simulink model "OMAP_ver_MIL10"  (R2018b)
settings: Solver=FixedStepDiscrete  StartTime=0.0  StopTime=10.0  FixedStep=0.01  RelTol=1e-3
undefined symbols (not defined in the file or in its folder): OMAP_Switch_EMS, OMAP_Switch_EPS, OMAP_Switch_ESC, OMAP_Switch_IC, OMAP_Switch_OTHER, TH_HMIClb_tiDgrdIconWarnHiDurT_C, TH_HMIClb_tiDgrdIconWarnLoDurT_C, TH_HMIClb_tiDgrdVocWarnDurT_C, TH_HMIClb_tiHndOffTxtWarnT_C, TH_HMIClb_tiHndOffVocWarnT_C, TH_HMIClb_tiSWALimFlgDetT_C, TH_HMIClb_tiTxtLimT_C
libraries: simulink x118
(part 4 of 9)

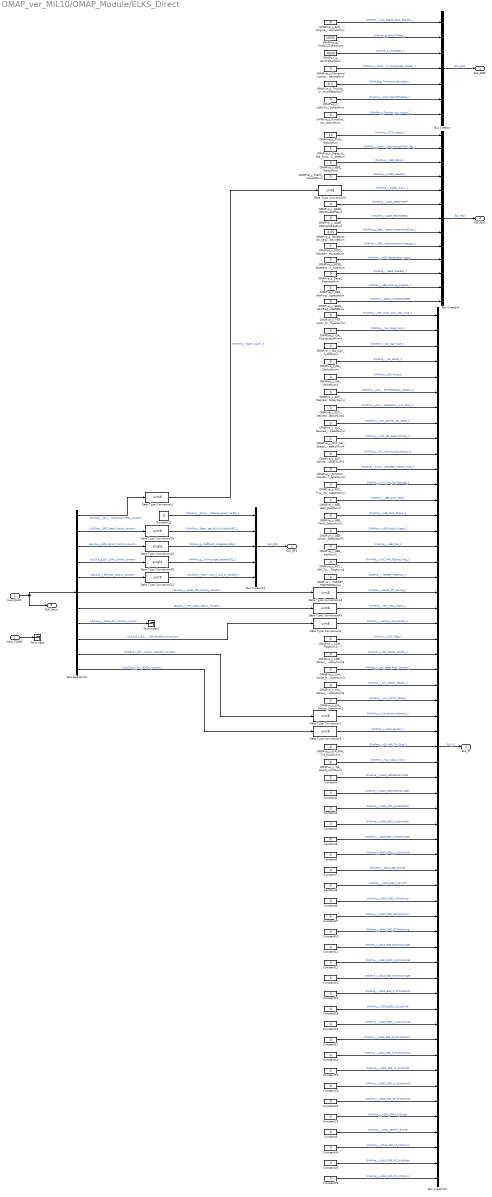
== system OMAP_ver_MIL10/OMAP_Module/ELKS_Direct ==
  Input_ELKS : Inport
  Input_FDMM : Inport  Port=2
  Bus Creator : BusCreator  Inputs=7
  Bus Creator13 : BusCreator  Inputs=5
  Bus Creator22 : BusCreator  Inputs=57
  Bus Creator5 : BusCreator  Inputs=13
  Bus Selector10 : BusSelector  OutputSignals=ELKSve_y_ELK_HapticAlarmReq_convert,ELKSve_y_EPS_State_Control_convert,ELKSve_g_EPS_Factor_Control_convert,ELKSve_g_ELK_SWA_Control_convert,ELKSve_y_EPS_ELK_Control_convert,ELKSve_y_Hands_Off_Warning_convert,ELKSve_y_HMI_Popup_Status_convert,ELKSve_y_state_ELK_function_convert,ELKSve_y_ELK_VehicleLaneDisp_convert,ELKSve_y_ELK_Action_Indication_convert,ELKSve_y_ELK_ELKSts_convert
  Constant{,1..27} (28 alike) : Constant  Value=0  OutDataTypeStr=uint8
  Data Type Conversion{1..5,28,31,44..45} (9 alike) : DataTypeConversion  OutDataTypeStr=uint8
  Data Type Conversion29 : DataTypeConversion  OutDataTypeStr=single
  Data Type Conversion30 : DataTypeConversion  OutDataTypeStr=single
  OMAPve_g_ACCTqReqNum : Constant  Value=-4000  OutDataTypeStr=single
  OMAPve_g_Deceleration_setpoint_deviceNum : Constant  Value=2.05  OutDataTypeStr=single
  OMAPve_g_PotACCTqReqNum : Constant  Value=-4000  OutDataTypeStr=single
  OMAPve_g_TminUp_or_downGearNum : Constant  Value=6.2  OutDataTypeStr=single
  OMAPve_y_ACC_DesiredHeadway_DisplayNum4 : Constant  Value=0  OutDataTypeStr=uint8
  OMAPve_y_ACC_DesiredHeadway_Icon_BasicNum4 : Constant  Value=0  OutDataTypeStr=uint8
  OMAPve_y_ACC_Desired_Set_SpeedNum4 : Constant  Value=0  OutDataTypeStr=uint8
  OMAPve_y_ACC_Engine_Start_RequestNum : Constant  Value=0  OutDataTypeStr=uint8
  OMAPve_y_ACC_HMI_TgtDisp_FlagNum4 : Constant  Value=0  OutDataTypeStr=uint8
  OMAPve_y_ACC_Pop_Up_MessageNum4 : Constant  Value=0  OutDataTypeStr=uint8
  OMAPve_y_ACC_Set_Speed_DisplayNum4 : Constant  Value=0  OutDataTypeStr=uint8
  OMAPve_y_ACC_Vehicle_Icon_DisplayNum4 : Constant  Value=0  OutDataTypeStr=uint8
  OMAPve_y_ADAS_ACCRequestEPBNum : Constant  Value=0  OutDataTypeStr=uint8
  OMAPve_y_ADAS_ESCDriveOffNum : Constant  Value=0  OutDataTypeStr=uint8
  OMAPve_y_ADAS_ESCHoldReqNum : Constant  Value=0  OutDataTypeStr=uint8
  OMAPve_y_AEB_Alert_ReqNum2 : Constant  Value=0  OutDataTypeStr=uint8
  OMAPve_y_AEB_Braking_progressNum : Constant  Value=0  OutDataTypeStr=uint8
  OMAPve_y_AEB_Fault_StatusNum2 : Constant  Value=0  OutDataTypeStr=uint8
  OMAPve_y_AEB_StatusNum : Constant  Value=5  OutDataTypeStr=uint8
  OMAPve_y_AEB_Switch_StatusNum2 : Constant  Value=0  OutDataTypeStr=uint8
  OMAPve_y_AEB_tipsNum2 : Constant  Value=0  OutDataTypeStr=uint8
  OMAPve_y_Decel_RequestNum : Constant  Value=0  OutDataTypeStr=uint8
  OMAPve_y_FCW_StatusNum : Constant  Value=10  OutDataTypeStr=uint8
  OMAPve_y_Function_Acc_statusNum : Constant  Value=3  OutDataTypeStr=uint8
  OMAPve_y_ICA_HMI_Txt_DispNum4 : Constant  Value=0  OutDataTypeStr=uint8
  OMAPve_y_ISA_Popup_textNum4 : Constant  Value=0  OutDataTypeStr=uint8
  OMAPve_y_ISA_Sign_TypeNum4 : Constant  Value=0  OutDataTypeStr=uint8
  OMAPve_y_ISA_StatusNum4 : Constant  Value=0  OutDataTypeStr=uint8
  OMAPve_y_ISA_ValueNum4 : Constant  Value=0  OutDataTypeStr=uint8
  OMAPve_y_LDW_FlagNum3 : Constant  Value=0  OutDataTypeStr=uint8
  OMAPve_y_LDW_Status_DisplayNum3 : Constant  Value=0  OutDataTypeStr=uint8
  OMAPve_y_LKA_Mode_from_CameraNum3 : Constant  Value=0  OutDataTypeStr=uint8
  OMAPve_y_LKA_Status_DisplayNum3 : Constant  Value=0  OutDataTypeStr=uint8
  OMAPve_y_LKA_Switch_StateNum3 : Constant  Value=0  OutDataTypeStr=uint8
  OMAPve_y_MDD_Decelerationcontrol_requestNum : Constant  Value=0  OutDataTypeStr=uint8
  OMAPve_y_MDD_deceleration_typeNum : Constant  Value=0  OutDataTypeStr=uint8
  OMAPve_y_Powertrain_torquewheel_requestNum : Constant  Value=0  OutDataTypeStr=uint8
  OMAPve_y_Prefill_requestNum : Constant  Value=0  OutDataTypeStr=uint8
  OMAPve_y_RVVACC_Vehiclespeed_request_typeNum4 : Constant  Value=0  OutDataTypeStr=uint8
  OMAPve_y_State_of_the_functionFARC_detNum : Constant  Value=5  OutDataTypeStr=uint8
  OMAPve_y_TARGET_POSITIONNum4 : Constant  Value=6  OutDataTypeStr=uint8
  OMAPve_y_TJA_status_iconNum4 : Constant  Value=0  OutDataTypeStr=uint8
  OMAPve_y_TSR_Vision_Only_Sign_TypeNum4 : Constant  Value=0  OutDataTypeStr=uint8
  OMAPve_y_stAcvTqWhlPTPotReqNum : Constant  Value=0  OutDataTypeStr=uint8
  Terminator : Terminator
  Terminator1 : Terminator
  ELK_EMS : Outport
  ELK_ESC : Outport  Port=2
  ELK_EPS : Outport  Port=3
  ELK_IC : Outport  Port=4
  ELK_Input : Outport  Port=5
  wires:
  Bus Creator22/1 -> ELK_IC/1  "ELK_IC"
  Data Type Conversion44/1 -> Bus Creator22/19  "OMAPve_y_Hands_off_warning_2"
  Data Type Conversion1/1 -> Bus Creator22/27  "OMAPve_y_LKA_action_indication_2"
  Bus Selector10/5 -> Data Type Conversion31/1  "<ELKSve_y_EPS_ELK_Control_convert>"
  Bus Selector10/2 -> Data Type Conversion28/1  "<ELKSve_y_EPS_State_Control_convert>"
  Data Type Conversion29/1 -> Bus Creator13/3  "OMAPve_g_Coefficient_toregulate_EPS_2"
  OMAPve_y_LDW_Status_DisplayNum3/1 -> Bus Creator22/23  "OMAPve_y_LDW_Status_Display_2"
  OMAPve_y_LDW_FlagNum3/1 -> Bus Creator22/22  "OMAPve_y_LDW_Flag_2"
  OMAPve_y_ACC_DesiredHeadway_Icon_BasicNum4/1 -> Bus Creator22/7  "OMAPve_y_ACC_DesiredHeadway_Icon_Basic_2"
  Bus Selector10/6 -> Data Type Conversion44/1  "<ELKSve_y_Hands_Off_Warning_convert>"
  Bus Selector10/4 -> Data Type Conversion30/1  "<ELKSve_g_ELK_SWA_Control_convert>"
  OMAPve_y_ACC_HMI_TgtDisp_FlagNum4/1 -> Bus Creator22/17  "OMAPve_y_ACC_HMI_TgtDisp_Flag_2"
  Bus Selector10/3 -> Data Type Conversion29/1  "<ELKSve_g_EPS_Factor_Control_convert>"
  Data Type Conversion4/1 -> Bus Creator22/21  "OMAPve_y_Vehicle_Lane_Display_2"
  OMAPve_y_TJA_status_iconNum4/1 -> Bus Creator22/30  "OMAPve_y_TJA_status_icon_2"
  Bus Selector10/8 -> Terminator1/1  "<ELKSve_y_state_ELK_function_convert>"
  OMAPve_y_TARGET_POSITIONNum4/1 -> Bus Creator22/18  "OMAPve_y_TARGET_POSITION_2"
  OMAPve_y_ACC_Vehicle_Icon_DisplayNum4/1 -> Bus Creator22/10  "OMAPve_y_ACC_Vehicle_Icon_Display_2"
  OMAPve_y_ACC_DesiredHeadway_DisplayNum4/1 -> Bus Creator22/6  "OMAPve_y_ACC_DesiredHeadway_Display_2"
  OMAPve_y_LKA_Status_DisplayNum3/1 -> Bus Creator22/25  "OMAPve_y_LKA_Status_Display_2"
  OMAPve_y_AEB_tipsNum2/1 -> Bus Creator22/16  "OMAPve_y_AEB_tips_2"
  OMAPve_y_ACC_Pop_Up_MessageNum4/1 -> Bus Creator22/12  "OMAPve_y_ACC_Pop_Up_Message_2"
  Bus Selector10/7 -> Data Type Conversion45/1  "<ELKSve_y_HMI_Popup_Status_convert>"
  OMAPve_y_ACC_Desired_Set_SpeedNum4/1 -> Bus Creator22/8  "OMAPve_y_ACC_Desired_Set_Speed_2"
  OMAPve_y_ICA_HMI_Txt_DispNum4/1 -> Bus Creator22/29  "OMAPve_y_ICA_HMI_Txt_Disp_2"
  Bus Creator13/1 -> ELK_EPS/1  "ELK_EPS"
  OMAPve_y_ISA_StatusNum4/1 -> Bus Creator22/4  "OMAPve_y_ISA_Status_2"
  OMAPve_y_ISA_Popup_textNum4/1 -> Bus Creator22/2  "OMAPve_y_ISA_Popup_text_2"
  OMAPve_y_AEB_Fault_StatusNum2/1 -> Bus Creator22/14  "OMAPve_y_AEB_Fault_Status_2"
  Data Type Conversion45/1 -> Bus Creator22/20  "OMAPve_y_HMI_Popup_Status_2"
  OMAPve_y_AEB_Switch_StatusNum2/1 -> Bus Creator22/15  "OMAPve_y_AEB_Switch_Status_2"
  OMAPve_y_LKA_Mode_from_CameraNum3/1 -> Bus Creator22/24  "OMAPve_y_LKA_Mode_from_Camera_2"
  OMAPve_y_AEB_Alert_ReqNum2/1 -> Bus Creator22/13  "OMAPve_y_AEB_Alert_Req_2"
  OMAPve_y_ACC_Set_Speed_DisplayNum4/1 -> Bus Creator22/9  "OMAPve_y_ACC_Set_Speed_Display_2"
  Input_ELKS/1 -> ELK_Input/1, Bus Selector10/1
  Constant23/1 -> Bus Creator13/1  "OMAPve_y_Power_steering_power_cut3F2_2"
  Data Type Conversion30/1 -> Bus Creator13/4  "OMAPve_g_Column_angle_setpoint3F2_2"
  OMAPve_y_ISA_ValueNum4/1 -> Bus Creator22/5  "OMAPve_y_ISA_Value_2"
  OMAPve_y_LKA_Switch_StateNum3/1 -> Bus Creator22/26  "OMAPve_y_LKA_Switch_State_2"
  Data Type Conversion28/1 -> Bus Creator13/2  "OMAPve_y_General_state_of_LKA_function3F2_2"
  Data Type Conversion31/1 -> Bus Creator13/5  "OMAPve_y_Permit_to_know_if_LKA_or_LPA3F2_2"
  OMAPve_y_RVVACC_Vehiclespeed_request_typeNum4/1 -> Bus Creator22/11  "OMAPve_y_RVVACC_Vehiclespeed_request_type_2"
  OMAPve_y_TSR_Vision_Only_Sign_TypeNum4/1 -> Bus Creator22/1  "OMAPve_y_TSR_Vision_Only_Sign_Type_2"
  OMAPve_y_ISA_Sign_TypeNum4/1 -> Bus Creator22/3  "OMAPve_y_ISA_Sign_Type_2"
  OMAPve_y_Function_Acc_statusNum/1 -> Bus Creator/7  "OMAPve_y_Function_Acc_status_1"
  OMAPve_y_stAcvTqWhlPTPotReqNum/1 -> Bus Creator/6  "OMAPve_y_stAcvTqWhlPTPotReq_1"
  Bus Creator/1 -> ELK_EMS/1  "ELK_EMS"
  OMAPve_y_ACC_Engine_Start_RequestNum/1 -> Bus Creator/1  "OMAPve_y_ACC_Engine_Start_Request_1"
  OMAPve_g_TminUp_or_downGearNum/1 -> Bus Creator/5  "OMAPve_g_TminUp_or_downGear_1"
  OMAPve_g_PotACCTqReqNum/1 -> Bus Creator/2  "OMAPve_g_PotACCTqReq_1"
  OMAPve_y_Powertrain_torquewheel_requestNum/1 -> Bus Creator/4  "OMAPve_y_Powertrain_torquewheel_request_1"
  OMAPve_g_ACCTqReqNum/1 -> Bus Creator/3  "OMAPve_g_ACCTqReq_1"
  OMAPve_g_Deceleration_setpoint_deviceNum/1 -> Bus Creator5/8  "OMAPve_g_Deceleration_setpoint_device_1"
  OMAPve_y_AEB_StatusNum/1 -> Bus Creator5/3  "OMAPve_y_AEB_Status_1"
  Data Type Conversion3/1 -> Bus Creator5/5  "OMAPve_y_Haptic_Alarm_1"
  OMAPve_y_AEB_Braking_progressNum/1 -> Bus Creator5/12  "OMAPve_y_AEB_Braking_progress_1"
  OMAPve_y_FCW_StatusNum/1 -> Bus Creator5/1  "OMAPve_y_FCW_Status_1"
  OMAPve_y_Decel_RequestNum/1 -> Bus Creator5/11  "OMAPve_y_Decel_Request_1"
  OMAPve_y_MDD_Decelerationcontrol_requestNum/1 -> Bus Creator5/9  "OMAPve_y_MDD_Decelerationcontrol_request_1"
  OMAPve_y_MDD_deceleration_typeNum/1 -> Bus Creator5/10  "OMAPve_y_MDD_deceleration_type_1"
  OMAPve_y_State_of_the_functionFARC_detNum/1 -> Bus Creator5/2  "OMAPve_y_State_of_the_functionFARC_det_1"
  OMAPve_y_Prefill_requestNum/1 -> Bus Creator5/4  "OMAPve_y_Prefill_request_1"
  Bus Creator5/1 -> ELK_ESC/1  "ELK_ESC"
  Input_FDMM/1 -> Terminator/1
  Bus Selector10/10 -> Data Type Conversion1/1  "<ELKSve_y_ELK_Action_Indication_convert>"
  Data Type Conversion2/1 -> Data Type Conversion3/1  "OMAPve_y_Haptic_Alarm_2"
  Bus Selector10/1 -> Data Type Conversion2/1  "<ELKSve_y_ELK_HapticAlarmReq_convert>"
  Bus Selector10/11 -> Data Type Conversion5/1  "<ELKSve_y_ELK_ELKSts_convert>"
  Bus Selector10/9 -> Data Type Conversion4/1  "<ELKSve_y_ELK_VehicleLaneDisp_convert>"
  Data Type Conversion5/1 -> Bus Creator22/28  "OMAPve_y_ADAS_ELKSts_2"
  OMAPve_y_ADAS_ESCHoldReqNum/1 -> Bus Creator5/7  "OMAPve_y_ADAS_ESCHoldReq"
  OMAPve_y_ADAS_ESCDriveOffNum/1 -> Bus Creator5/6  "OMAPve_y_ADAS_ESCDriveOff"
  OMAPve_y_ADAS_ACCRequestEPBNum/1 -> Bus Creator5/13  "OMAPve_y_ADAS_ACCRequestEPB"
  Constant17/1 -> Bus Creator22/48  "OMAPve_y_ADAS_BSD_S_DoorOpenWrn"
  Constant16/1 -> Bus Creator22/47  "OMAPve_y_ADAS_BSD_S_LCAWarning"
  Constant1/1 -> Bus Creator22/32  "OMAPve_y_ADAS_RighrLEDWarningSt"
  Constant19/1 -> Bus Creator22/50  "OMAPve_y_ADAS_SRR_LF_SystStInfo"
  Constant10/1 -> Bus Creator22/41  "OMAPve_y_ADAS_BSD_RCTAWarning"
  Constant27/1 -> Bus Creator22/40  "OMAPve_y_ADAS_BSD_DoorOpenWrn"
  Constant22/1 -> Bus Creator22/53  "OMAPve_y_ADAS_SRR-LF_ErrorSt"
  Constant18/1 -> Bus Creator22/49  "OMAPve_y_ADAS_BSD_S_RCTAWarning"
  Constant20/1 -> Bus Creator22/51  "OMAPve_y_ADAS_SRR_LF_SystWorkSt"
  Constant21/1 -> Bus Creator22/52  "OMAPve_y_ADAS_SRR_RF_SystWorkSt"
  Constant15/1 -> Bus Creator22/46  "OMAPve_y_ADAS_BSD_S_SystStInfo"
  Constant14/1 -> Bus Creator22/45  "OMAPve_y_ADAS_BSD_S_RCTAWorkSt"
  Constant13/1 -> Bus Creator22/44  "OMAPve_y_ADAS_BSD_RCTAWorkingSt"
  Constant3/1 -> Bus Creator22/54  "OMAPve_y_ADAS_SRR-RF_ErrorSt"
  Constant26/1 -> Bus Creator22/57  "OMAPve_y_ADAS_SRR_RF_FCTAWrn"
  Constant/1 -> Bus Creator22/31  "OMAPve_y_ADAS_LeftLEDWarningSt"
  Constant25/1 -> Bus Creator22/56  "OMAPve_y_ADAS_SRR_RF_SystStInfo"
  Constant24/1 -> Bus Creator22/55  "OMAPve_y_ADAS_SRR_LF_FCTAWrn"
  Constant5/1 -> Bus Creator22/35  "OMAPve_y_ADAS_BSD_LCWWorkingSt"
  Constant9/1 -> Bus Creator22/39  "OMAPve_y_ADAS_BSD_LCAWarning"
  Constant12/1 -> Bus Creator22/43  "OMAPve_y_ADAS_BSD_S_DOWWorkSt"
  Constant6/1 -> Bus Creator22/36  "OMAPve_y_ADAS_BSD_S_LCWWorkSt"
  Constant8/1 -> Bus Creator22/38  "OMAPve_y_ADAS_BSD_S_ErrorSt"
  Constant2/1 -> Bus Creator22/33  "OMAPve_y_ADAS_SRR_SystemState"
  Constant7/1 -> Bus Creator22/37  "OMAPve_y_ADAS_BSD_ErrorSt"
  Constant4/1 -> Bus Creator22/34  "OMAPve_y_ADAS_BSD_SystemStInfo"
  Constant11/1 -> Bus Creator22/42  "OMAPve_y_ADAS_BSD_DOWWorkingSt"

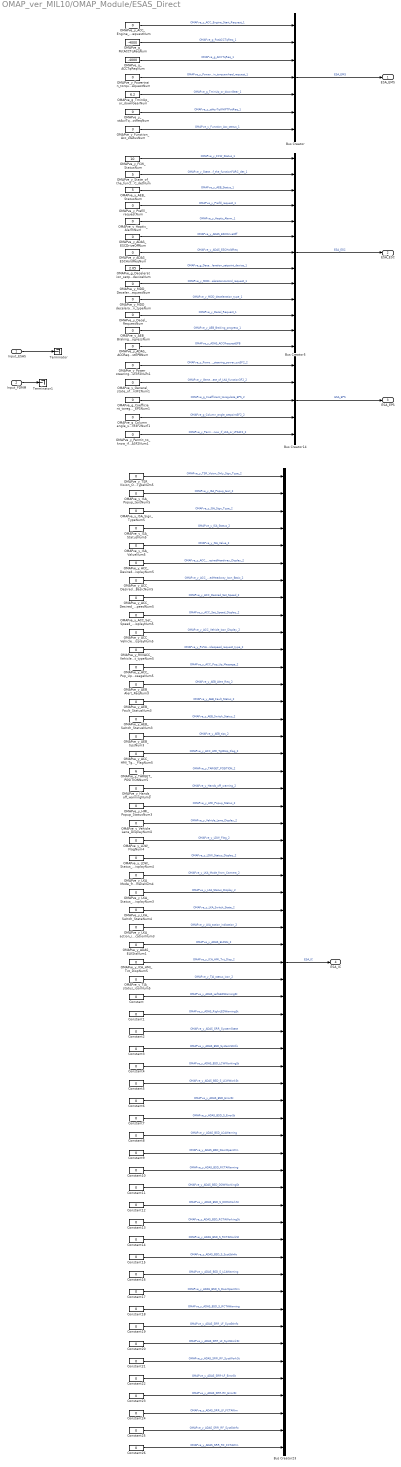
== system OMAP_ver_MIL10/OMAP_Module/ESAS_Direct ==
  Input_ESAS : Inport
  Input_FDMM : Inport  Port=2
  Bus Creator : BusCreator  Inputs=7
  Bus Creator14 : BusCreator  Inputs=5
  Bus Creator23 : BusCreator  Inputs=57
  Bus Creator5 : BusCreator  Inputs=13
  Constant{,1..26} (27 alike) : Constant  Value=0  OutDataTypeStr=uint8
  OMAPve_g_ACCTqReqNum : Constant  Value=-4000  OutDataTypeStr=single
  OMAPve_g_Coefficient_toregulate_EPSNum1 : Constant  Value=0  OutDataTypeStr=single
  OMAPve_g_Column_angle_setpoint3F2Num1 : Constant  Value=0  OutDataTypeStr=single
  OMAPve_g_Deceleration_setpoint_deviceNum : Constant  Value=2.05  OutDataTypeStr=single
  OMAPve_g_PotACCTqReqNum : Constant  Value=-4000  OutDataTypeStr=single
  OMAPve_g_TminUp_or_downGearNum : Constant  Value=6.2  OutDataTypeStr=single
  OMAPve_y_ACC_DesiredHeadway_DisplayNum5 : Constant  Value=0  OutDataTypeStr=uint8
  OMAPve_y_ACC_DesiredHeadway_Icon_BasicNum5 : Constant  Value=0  OutDataTypeStr=uint8
  OMAPve_y_ACC_Desired_Set_SpeedNum5 : Constant  Value=0  OutDataTypeStr=uint8
  OMAPve_y_ACC_Engine_Start_RequestNum : Constant  Value=0  OutDataTypeStr=uint8
  OMAPve_y_ACC_HMI_TgtDisp_FlagNum5 : Constant  Value=0  OutDataTypeStr=uint8
  OMAPve_y_ACC_Pop_Up_MessageNum5 : Constant  Value=0  OutDataTypeStr=uint8
  OMAPve_y_ACC_Set_Speed_DisplayNum5 : Constant  Value=0  OutDataTypeStr=uint8
  OMAPve_y_ACC_Vehicle_Icon_DisplayNum5 : Constant  Value=0  OutDataTypeStr=uint8
  OMAPve_y_ADAS_ACCRequestEPBNum : Constant  Value=0  OutDataTypeStr=uint8
  OMAPve_y_ADAS_ELKStsNum1 : Constant  Value=0  OutDataTypeStr=uint8
  OMAPve_y_ADAS_ESCDriveOffNum : Constant  Value=0  OutDataTypeStr=uint8
  OMAPve_y_ADAS_ESCHoldReqNum : Constant  Value=0  OutDataTypeStr=uint8
  OMAPve_y_AEB_Alert_ReqNum3 : Constant  Value=0  OutDataTypeStr=uint8
  OMAPve_y_AEB_Braking_progressNum : Constant  Value=0  OutDataTypeStr=uint8
  OMAPve_y_AEB_Fault_StatusNum3 : Constant  Value=0  OutDataTypeStr=uint8
  OMAPve_y_AEB_StatusNum : Constant  Value=5  OutDataTypeStr=uint8
  OMAPve_y_AEB_Switch_StatusNum3 : Constant  Value=0  OutDataTypeStr=uint8
  OMAPve_y_AEB_tipsNum3 : Constant  Value=0  OutDataTypeStr=uint8
  OMAPve_y_Decel_RequestNum : Constant  Value=0  OutDataTypeStr=uint8
  OMAPve_y_FCW_StatusNum : Constant  Value=10  OutDataTypeStr=uint8
  OMAPve_y_Function_Acc_statusNum : Constant  Value=3  OutDataTypeStr=uint8
  OMAPve_y_General_state_of_LKA_function3F2Num1 : Constant  Value=0  OutDataTypeStr=uint8
  OMAPve_y_HMI_Popup_StatusNum3 : Constant  Value=0  OutDataTypeStr=uint8
  OMAPve_y_Hands_off_warningNum3 : Constant  Value=0  OutDataTypeStr=uint8
  OMAPve_y_Haptic_AlarmNum : Constant  Value=0  OutDataTypeStr=uint8
  OMAPve_y_ICA_HMI_Txt_DispNum5 : Constant  Value=0  OutDataTypeStr=uint8
  OMAPve_y_ISA_Popup_textNum5 : Constant  Value=0  OutDataTypeStr=uint8
  OMAPve_y_ISA_Sign_TypeNum5 : Constant  Value=0  OutDataTypeStr=uint8
  OMAPve_y_ISA_StatusNum5 : Constant  Value=0  OutDataTypeStr=uint8
  OMAPve_y_ISA_ValueNum5 : Constant  Value=0  OutDataTypeStr=uint8
  OMAPve_y_LDW_FlagNum4 : Constant  Value=0  OutDataTypeStr=uint8
  OMAPve_y_LDW_Status_DisplayNum4 : Constant  Value=0  OutDataTypeStr=uint8
  OMAPve_y_LKA_Mode_from_CameraNum4 : Constant  Value=0  OutDataTypeStr=uint8
  OMAPve_y_LKA_Status_DisplayNum3 : Constant  Value=0  OutDataTypeStr=uint8
  OMAPve_y_LKA_Switch_StateNum4 : Constant  Value=0  OutDataTypeStr=uint8
  OMAPve_y_LKA_action_indicationNum3 : Constant  Value=0  OutDataTypeStr=uint8
  OMAPve_y_MDD_Decelerationcontrol_requestNum : Constant  Value=0  OutDataTypeStr=uint8
  OMAPve_y_MDD_deceleration_typeNum : Constant  Value=0  OutDataTypeStr=uint8
  OMAPve_y_Permit_to_know_if_LKA_or_LPA3F2Num1 : Constant  Value=0  OutDataTypeStr=uint8
  OMAPve_y_Power_steering_power_cut3F2Num1 : Constant  Value=0  OutDataTypeStr=uint8
  OMAPve_y_Powertrain_torquewheel_requestNum : Constant  Value=0  OutDataTypeStr=uint8
  OMAPve_y_Prefill_requestNum : Constant  Value=0  OutDataTypeStr=uint8
  OMAPve_y_RVVACC_Vehiclespeed_request_typeNum5 : Constant  Value=0  OutDataTypeStr=uint8
  OMAPve_y_State_of_the_functionFARC_detNum : Constant  Value=5  OutDataTypeStr=uint8
  OMAPve_y_TARGET_POSITIONNum5 : Constant  Value=6  OutDataTypeStr=uint8
  OMAPve_y_TJA_status_iconNum5 : Constant  Value=0  OutDataTypeStr=uint8
  OMAPve_y_TSR_Vision_Only_Sign_TypeNum5 : Constant  Value=0  OutDataTypeStr=uint8
  OMAPve_y_Vehicle_Lane_DisplayNum4 : Constant  Value=0  OutDataTypeStr=uint8
  OMAPve_y_stAcvTqWhlPTPotReqNum : Constant  Value=0  OutDataTypeStr=uint8
  Terminator : Terminator
  Terminator1 : Terminator
  ESA_EMS : Outport
  ESA_ESC : Outport  Port=2
  ESA_EPS : Outport  Port=3
  ESA_IC : Outport  Port=4
  wires:
  Bus Creator23/1 -> ESA_IC/1  "ESA_IC"
  Bus Creator14/1 -> ESA_EPS/1  "ESA_EPS"
  OMAPve_y_AEB_Fault_StatusNum3/1 -> Bus Creator23/14  "OMAPve_y_AEB_Fault_Status_2"
  OMAPve_y_ISA_Sign_TypeNum5/1 -> Bus Creator23/3  "OMAPve_y_ISA_Sign_Type_2"
  OMAPve_y_ACC_Vehicle_Icon_DisplayNum5/1 -> Bus Creator23/10  "OMAPve_y_ACC_Vehicle_Icon_Display_2"
  OMAPve_y_TSR_Vision_Only_Sign_TypeNum5/1 -> Bus Creator23/1  "OMAPve_y_TSR_Vision_Only_Sign_Type_2"
  OMAPve_y_AEB_Alert_ReqNum3/1 -> Bus Creator23/13  "OMAPve_y_AEB_Alert_Req_2"
  OMAPve_y_TJA_status_iconNum5/1 -> Bus Creator23/30  "OMAPve_y_TJA_status_icon_2"
  OMAPve_y_TARGET_POSITIONNum5/1 -> Bus Creator23/18  "OMAPve_y_TARGET_POSITION_2"
  OMAPve_y_AEB_Switch_StatusNum3/1 -> Bus Creator23/15  "OMAPve_y_AEB_Switch_Status_2"
  OMAPve_y_AEB_tipsNum3/1 -> Bus Creator23/16  "OMAPve_y_AEB_tips_2"
  OMAPve_y_ICA_HMI_Txt_DispNum5/1 -> Bus Creator23/29  "OMAPve_y_ICA_HMI_Txt_Disp_2"
  OMAPve_y_ACC_Desired_Set_SpeedNum5/1 -> Bus Creator23/8  "OMAPve_y_ACC_Desired_Set_Speed_2"
  OMAPve_y_ACC_DesiredHeadway_DisplayNum5/1 -> Bus Creator23/6  "OMAPve_y_ACC_DesiredHeadway_Display_2"
  OMAPve_y_LKA_Switch_StateNum4/1 -> Bus Creator23/26  "OMAPve_y_LKA_Switch_State_2"
  Input_ESAS/1 -> Terminator/1
  OMAPve_y_LKA_Status_DisplayNum3/1 -> Bus Creator23/25  "OMAPve_y_LKA_Status_Display_2"
  OMAPve_y_LDW_Status_DisplayNum4/1 -> Bus Creator23/23  "OMAPve_y_LDW_Status_Display_2"
  OMAPve_y_ACC_Pop_Up_MessageNum5/1 -> Bus Creator23/12  "OMAPve_y_ACC_Pop_Up_Message_2"
  OMAPve_y_ACC_Set_Speed_DisplayNum5/1 -> Bus Creator23/9  "OMAPve_y_ACC_Set_Speed_Display_2"
  OMAPve_g_Column_angle_setpoint3F2Num1/1 -> Bus Creator14/4  "OMAPve_g_Column_angle_setpoint3F2_2"
  OMAPve_y_HMI_Popup_StatusNum3/1 -> Bus Creator23/20  "OMAPve_y_HMI_Popup_Status_2"
  OMAPve_y_Vehicle_Lane_DisplayNum4/1 -> Bus Creator23/21  "OMAPve_y_Vehicle_Lane_Display_2"
  OMAPve_y_ACC_HMI_TgtDisp_FlagNum5/1 -> Bus Creator23/17  "OMAPve_y_ACC_HMI_TgtDisp_Flag_2"
  OMAPve_g_Coefficient_toregulate_EPSNum1/1 -> Bus Creator14/3  "OMAPve_g_Coefficient_toregulate_EPS_2"
  OMAPve_y_ISA_StatusNum5/1 -> Bus Creator23/4  "OMAPve_y_ISA_Status_2"
  OMAPve_y_ISA_Popup_textNum5/1 -> Bus Creator23/2  "OMAPve_y_ISA_Popup_text_2"
  OMAPve_y_ISA_ValueNum5/1 -> Bus Creator23/5  "OMAPve_y_ISA_Value_2"
  OMAPve_y_Hands_off_warningNum3/1 -> Bus Creator23/19  "OMAPve_y_Hands_off_warning_2"
  OMAPve_y_LKA_action_indicationNum3/1 -> Bus Creator23/27  "OMAPve_y_LKA_action_indication_2"
  OMAPve_y_LKA_Mode_from_CameraNum4/1 -> Bus Creator23/24  "OMAPve_y_LKA_Mode_from_Camera_2"
  OMAPve_y_General_state_of_LKA_function3F2Num1/1 -> Bus Creator14/2  "OMAPve_y_General_state_of_LKA_function3F2_2"
  OMAPve_y_RVVACC_Vehiclespeed_request_typeNum5/1 -> Bus Creator23/11  "OMAPve_y_RVVACC_Vehiclespeed_request_type_2"
  OMAPve_y_Permit_to_know_if_LKA_or_LPA3F2Num1/1 -> Bus Creator14/5  "OMAPve_y_Permit_to_know_if_LKA_or_LPA3F2_2"
  OMAPve_y_LDW_FlagNum4/1 -> Bus Creator23/22  "OMAPve_y_LDW_Flag_2"
  OMAPve_y_Power_steering_power_cut3F2Num1/1 -> Bus Creator14/1  "OMAPve_y_Power_steering_power_cut3F2_2"
  OMAPve_y_ACC_DesiredHeadway_Icon_BasicNum5/1 -> Bus Creator23/7  "OMAPve_y_ACC_DesiredHeadway_Icon_Basic_2"
  OMAPve_y_State_of_the_functionFARC_detNum/1 -> Bus Creator5/2  "OMAPve_y_State_of_the_functionFARC_det_1"
  OMAPve_y_Haptic_AlarmNum/1 -> Bus Creator5/5  "OMAPve_y_Haptic_Alarm_1"
  OMAPve_y_FCW_StatusNum/1 -> Bus Creator5/1  "OMAPve_y_FCW_Status_1"
  OMAPve_y_MDD_deceleration_typeNum/1 -> Bus Creator5/10  "OMAPve_y_MDD_deceleration_type_1"
  Bus Creator5/1 -> ESA_ESC/1  "ESA_ESC"
  OMAPve_y_MDD_Decelerationcontrol_requestNum/1 -> Bus Creator5/9  "OMAPve_y_MDD_Decelerationcontrol_request_1"
  OMAPve_y_AEB_Braking_progressNum/1 -> Bus Creator5/12  "OMAPve_y_AEB_Braking_progress_1"
  OMAPve_y_AEB_StatusNum/1 -> Bus Creator5/3  "OMAPve_y_AEB_Status_1"
  OMAPve_g_Deceleration_setpoint_deviceNum/1 -> Bus Creator5/8  "OMAPve_g_Deceleration_setpoint_device_1"
  OMAPve_g_ACCTqReqNum/1 -> Bus Creator/3  "OMAPve_g_ACCTqReq_1"
  Bus Creator/1 -> ESA_EMS/1  "ESA_EMS"
  OMAPve_g_PotACCTqReqNum/1 -> Bus Creator/2  "OMAPve_g_PotACCTqReq_1"
  OMAPve_y_ACC_Engine_Start_RequestNum/1 -> Bus Creator/1  "OMAPve_y_ACC_Engine_Start_Request_1"
  OMAPve_y_stAcvTqWhlPTPotReqNum/1 -> Bus Creator/6  "OMAPve_y_stAcvTqWhlPTPotReq_1"
  OMAPve_y_Decel_RequestNum/1 -> Bus Creator5/11  "OMAPve_y_Decel_Request_1"
  OMAPve_y_Function_Acc_statusNum/1 -> Bus Creator/7  "OMAPve_y_Function_Acc_status_1"
  OMAPve_g_TminUp_or_downGearNum/1 -> Bus Creator/5  "OMAPve_g_TminUp_or_downGear_1"
  OMAPve_y_Prefill_requestNum/1 -> Bus Creator5/4  "OMAPve_y_Prefill_request_1"
  OMAPve_y_Powertrain_torquewheel_requestNum/1 -> Bus Creator/4  "OMAPve_y_Powertrain_torquewheel_request_1"
  Input_FDMM/1 -> Terminator1/1
  OMAPve_y_ADAS_ELKStsNum1/1 -> Bus Creator23/28  "OMAPve_y_ADAS_ELKSts_2"
  OMAPve_y_ADAS_ESCHoldReqNum/1 -> Bus Creator5/7  "OMAPve_y_ADAS_ESCHoldReq"
  OMAPve_y_ADAS_ESCDriveOffNum/1 -> Bus Creator5/6  "OMAPve_y_ADAS_ESCDriveOff"
  OMAPve_y_ADAS_ACCRequestEPBNum/1 -> Bus Creator5/13  "OMAPve_y_ADAS_ACCRequestEPB"
  Constant18/1 -> Bus Creator23/49  "OMAPve_y_ADAS_BSD_S_RCTAWarning"
  Constant5/1 -> Bus Creator23/36  "OMAPve_y_ADAS_BSD_S_LCWWorkSt"
  Constant4/1 -> Bus Creator23/35  "OMAPve_y_ADAS_BSD_LCWWorkingSt"
  Constant10/1 -> Bus Creator23/41  "OMAPve_y_ADAS_BSD_RCTAWarning"
  Constant6/1 -> Bus Creator23/37  "OMAPve_y_ADAS_BSD_ErrorSt"
  Constant22/1 -> Bus Creator23/53  "OMAPve_y_ADAS_SRR-LF_ErrorSt"
  Constant13/1 -> Bus Creator23/44  "OMAPve_y_ADAS_BSD_RCTAWorkingSt"
  Constant17/1 -> Bus Creator23/48  "OMAPve_y_ADAS_BSD_S_DoorOpenWrn"
  Constant3/1 -> Bus Creator23/34  "OMAPve_y_ADAS_BSD_SystemStInfo"
  Constant23/1 -> Bus Creator23/54  "OMAPve_y_ADAS_SRR-RF_ErrorSt"
  Constant/1 -> Bus Creator23/31  "OMAPve_y_ADAS_LeftLEDWarningSt"
  Constant7/1 -> Bus Creator23/38  "OMAPve_y_ADAS_BSD_S_ErrorSt"
  Constant16/1 -> Bus Creator23/47  "OMAPve_y_ADAS_BSD_S_LCAWarning"
  Constant15/1 -> Bus Creator23/46  "OMAPve_y_ADAS_BSD_S_SystStInfo"
  Constant12/1 -> Bus Creator23/43  "OMAPve_y_ADAS_BSD_S_DOWWorkSt"
  Constant11/1 -> Bus Creator23/42  "OMAPve_y_ADAS_BSD_DOWWorkingSt"
  Constant20/1 -> Bus Creator23/51  "OMAPve_y_ADAS_SRR_LF_SystWorkSt"
  Constant25/1 -> Bus Creator23/56  "OMAPve_y_ADAS_SRR_RF_SystStInfo"
  Constant2/1 -> Bus Creator23/33  "OMAPve_y_ADAS_SRR_SystemState"
  Constant24/1 -> Bus Creator23/55  "OMAPve_y_ADAS_SRR_LF_FCTAWrn"
  Constant26/1 -> Bus Creator23/57  "OMAPve_y_ADAS_SRR_RF_FCTAWrn"
  Constant1/1 -> Bus Creator23/32  "OMAPve_y_ADAS_RighrLEDWarningSt"
  Constant8/1 -> Bus Creator23/39  "OMAPve_y_ADAS_BSD_LCAWarning"
  Constant14/1 -> Bus Creator23/45  "OMAPve_y_ADAS_BSD_S_RCTAWorkSt"
  Constant9/1 -> Bus Creator23/40  "OMAPve_y_ADAS_BSD_DoorOpenWrn"
  Constant19/1 -> Bus Creator23/50  "OMAPve_y_ADAS_SRR_LF_SystStInfo"
  Constant21/1 -> Bus Creator23/52  "OMAPve_y_ADAS_SRR_RF_SystWorkSt"

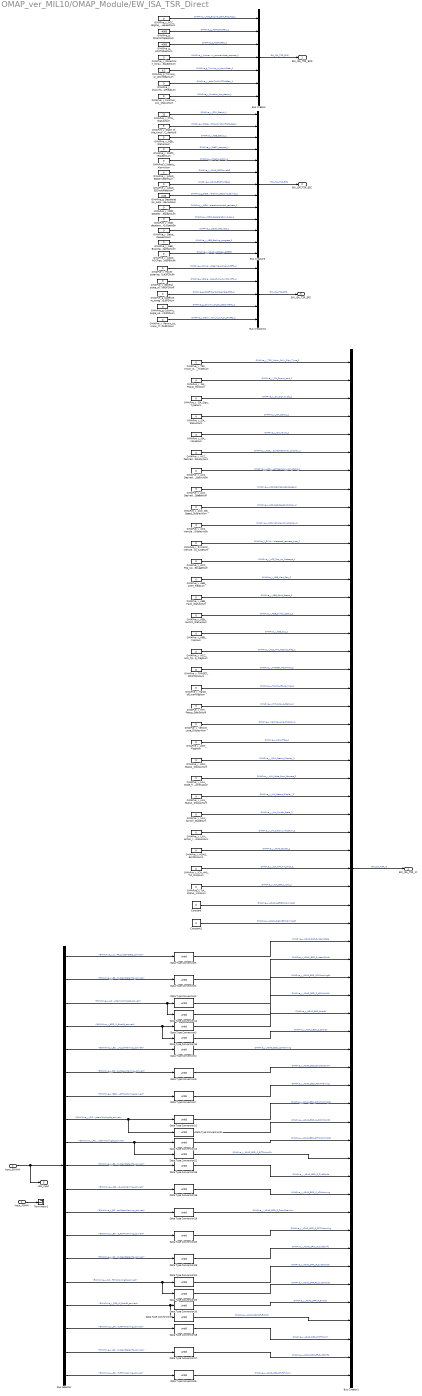
== system OMAP_ver_MIL10/OMAP_Module/EW_ISA_TSR_Direct ==
  Input_EWWW : Inport
  Input_FDMM : Inport  Port=2
  Bus Creator : BusCreator  Inputs=7
  Bus Creator1 : BusCreator  Inputs=57
  Bus Creator10 : BusCreator  Inputs=5
  Bus Creator5 : BusCreator  Inputs=13
  Bus Selector : BusSelector  OutputSignals=EWWWve_y_SRR_SystemState_convert,EWWWve_y_BSD_SystemStateInfo_convert,EWWWve_y_LCW_M_SystemWorkingSt_convert,EWWWve_y_BSD_M_ErrorSt_convert,EWWWve_y_BSD_M_LCAWarning_convert,EWWWve_y_BSD_M_DoorOpenWarning_convert,EWWWve_y_BSD_M_RCTAWarning_convert,EWWWve_y_DOW_M_SystemWorkingSt_convert,EWWWve_y_RCTA_M_SystemWorkingSt_convert,EWWWve_y_BSD_S_SystemStateInfo_convert,EWWWve_y_BSD_S_LCAWarning_convert,EWWWve_y_BSD_S_DoorOpenWarning_convert,EWWWve_y_BSD_S_RCTAWarning_convert,EWWWve_y_SRR_LF_SystemStateInfo_convert,EWWWve_y_SRR_LF_FCTAWorkingSt_convert,EWWWve_y_SRR_LF_ErrorSt_convert,EWWWve_y_SRR_LF_FCTAWarning_convert,EWWWve_y_SRR_RF_SystemStateInfo_convert,EWWWve_y_SRR_RF_FCTAWarning_convert
  Constant : Constant  Value=0  OutDataTypeStr=uint8
  Constant1 : Constant  Value=0  OutDataTypeStr=uint8
  Data Type Conversion{1..25} (25 alike) : DataTypeConversion  OutDataTypeStr=uint8
  OMAPve_g_ACCTqReqNum : Constant  Value=-4000  OutDataTypeStr=single
  OMAPve_g_Coefficient_toregulate_EPSNum : Constant  Value=0  OutDataTypeStr=single
  OMAPve_g_Column_angle_setpoint3F2Num : Constant  Value=0  OutDataTypeStr=single
  OMAPve_g_Deceleration_setpoint_deviceNum : Constant  Value=2.05  OutDataTypeStr=single
  OMAPve_g_PotACCTqReqNum : Constant  Value=-4000  OutDataTypeStr=single
  OMAPve_g_TminUp_or_downGearNum : Constant  Value=6.2  OutDataTypeStr=single
  OMAPve_y_ACC_DesiredHeadway_DisplayNum : Constant  Value=0  OutDataTypeStr=uint8
  OMAPve_y_ACC_DesiredHeadway_Icon_BasicNum : Constant  Value=0  OutDataTypeStr=uint8
  OMAPve_y_ACC_Desired_Set_SpeedNum : Constant  Value=0  OutDataTypeStr=uint8
  OMAPve_y_ACC_Engine_Start_RequestNum : Constant  Value=0  OutDataTypeStr=uint8
  OMAPve_y_ACC_HMI_TgtDisp_FlagNum : Constant  Value=0  OutDataTypeStr=uint8
  OMAPve_y_ACC_Pop_Up_MessageNum : Constant  Value=0  OutDataTypeStr=uint8
  OMAPve_y_ACC_Set_Speed_DisplayNum : Constant  Value=0  OutDataTypeStr=uint8
  OMAPve_y_ACC_Vehicle_Icon_DisplayNum : Constant  Value=0  OutDataTypeStr=uint8
  OMAPve_y_ADAS_ACCRequestEPBNum : Constant  Value=0  OutDataTypeStr=uint8
  OMAPve_y_ADAS_ELKStsNum1 : Constant  Value=0  OutDataTypeStr=uint8
  OMAPve_y_ADAS_ESCDriveOffNum : Constant  Value=0  OutDataTypeStr=uint8
  OMAPve_y_ADAS_ESCHoldReqNum : Constant  Value=0  OutDataTypeStr=uint8
  OMAPve_y_AEB_Alert_ReqNum : Constant  Value=0  OutDataTypeStr=uint8
  OMAPve_y_AEB_Braking_progressNum : Constant  Value=0  OutDataTypeStr=uint8
  OMAPve_y_AEB_Fault_StatusNum : Constant  Value=0  OutDataTypeStr=uint8
  OMAPve_y_AEB_StatusNum : Constant  Value=5  OutDataTypeStr=uint8
  OMAPve_y_AEB_Switch_StatusNum : Constant  Value=0  OutDataTypeStr=uint8
  OMAPve_y_AEB_tipsNum : Constant  Value=0  OutDataTypeStr=uint8
  OMAPve_y_Decel_RequestNum : Constant  Value=0  OutDataTypeStr=uint8
  OMAPve_y_FCW_StatusNum : Constant  Value=10  OutDataTypeStr=uint8
  OMAPve_y_Function_Acc_statusNum : Constant  Value=3  OutDataTypeStr=uint8
  OMAPve_y_General_state_of_LKA_function3F2Num : Constant  Value=0  OutDataTypeStr=uint8
  OMAPve_y_HMI_Popup_StatusNum : Constant  Value=0  OutDataTypeStr=uint8
  OMAPve_y_Hands_off_warningNum : Constant  Value=0  OutDataTypeStr=uint8
  OMAPve_y_Haptic_AlarmNum : Constant  Value=0  OutDataTypeStr=uint8
  OMAPve_y_ICA_HMI_Txt_DispNum : Constant  Value=0  OutDataTypeStr=uint8
  OMAPve_y_ISA_Popup_textNum : Constant  Value=0  OutDataTypeStr=uint8
  OMAPve_y_ISA_Sign_TypeNum : Constant  Value=0  OutDataTypeStr=uint8
  OMAPve_y_ISA_StatusNum : Constant  Value=0  OutDataTypeStr=uint8
  OMAPve_y_ISA_ValueNum : Constant  Value=0  OutDataTypeStr=uint8
  OMAPve_y_LDW_FlagNum : Constant  Value=0  OutDataTypeStr=uint8
  OMAPve_y_LDW_Status_DisplayNum : Constant  Value=0  OutDataTypeStr=uint8
  OMAPve_y_LKA_Mode_from_CameraNum : Constant  Value=0  OutDataTypeStr=uint8
  OMAPve_y_LKA_Status_DisplayNum : Constant  Value=0  OutDataTypeStr=uint8
  OMAPve_y_LKA_Switch_StateNum : Constant  Value=0  OutDataTypeStr=uint8
  OMAPve_y_LKA_action_indicationNum : Constant  Value=0  OutDataTypeStr=uint8
  OMAPve_y_MDD_Decelerationcontrol_requestNum : Constant  Value=0  OutDataTypeStr=uint8
  OMAPve_y_MDD_deceleration_typeNum : Constant  Value=0  OutDataTypeStr=uint8
  OMAPve_y_Permit_to_know_if_LKA_or_LPA3F2Num : Constant  Value=0  OutDataTypeStr=uint8
  OMAPve_y_Power_steering_power_cut3F2Num : Constant  Value=0  OutDataTypeStr=uint8
  OMAPve_y_Powertrain_torquewheel_requestNum : Constant  Value=0  OutDataTypeStr=uint8
  OMAPve_y_Prefill_requestNum : Constant  Value=0  OutDataTypeStr=uint8
  OMAPve_y_RVVACC_Vehiclespeed_request_typeNum : Constant  Value=0  OutDataTypeStr=uint8
  OMAPve_y_State_of_the_functionFARC_detNum : Constant  Value=5  OutDataTypeStr=uint8
  OMAPve_y_TARGET_POSITIONNum : Constant  Value=6  OutDataTypeStr=uint8
  OMAPve_y_TJA_status_iconNum : Constant  Value=0  OutDataTypeStr=uint8
  OMAPve_y_TSR_Vision_Only_Sign_TypeNum : Constant  Value=0  OutDataTypeStr=uint8
  OMAPve_y_Vehicle_Lane_DisplayNum : Constant  Value=0  OutDataTypeStr=uint8
  OMAPve_y_stAcvTqWhlPTPotReqNum : Constant  Value=0  OutDataTypeStr=uint8
  Terminator1 : Terminator
  EW_ISA_TSR_EMS : Outport
  EW_ISA_TSR_ESC : Outport  Port=2
  EW_ISA_TSR_EPS : Outport  Port=3
  EW_ISA_TSR_IC : Outport  Port=4
  EW_Input : Outport  Port=5
  wires:
  Bus Creator1/1 -> EW_ISA_TSR_IC/1  "EW_ISA_TSR_IC"
  Input_EWWW/1 -> EW_Input/1, Bus Selector/1
  Input_FDMM/1 -> Terminator1/1
  OMAPve_y_ACC_Engine_Start_RequestNum/1 -> Bus Creator/1  "OMAPve_y_ACC_Engine_Start_Request_1"
  OMAPve_y_Function_Acc_statusNum/1 -> Bus Creator/7  "OMAPve_y_Function_Acc_status_1"
  OMAPve_g_ACCTqReqNum/1 -> Bus Creator/3  "OMAPve_g_ACCTqReq_1"
  OMAPve_g_TminUp_or_downGearNum/1 -> Bus Creator/5  "OMAPve_g_TminUp_or_downGear_1"
  OMAPve_g_PotACCTqReqNum/1 -> Bus Creator/2  "OMAPve_g_PotACCTqReq_1"
  OMAPve_y_AEB_StatusNum/1 -> Bus Creator5/3  "OMAPve_y_AEB_Status_1"
  OMAPve_g_Deceleration_setpoint_deviceNum/1 -> Bus Creator5/8  "OMAPve_g_Deceleration_setpoint_device_1"
  OMAPve_y_Prefill_requestNum/1 -> Bus Creator5/4  "OMAPve_y_Prefill_request_1"
  OMAPve_y_Haptic_AlarmNum/1 -> Bus Creator5/5  "OMAPve_y_Haptic_Alarm_1"
  OMAPve_y_FCW_StatusNum/1 -> Bus Creator5/1  "OMAPve_y_FCW_Status_1"
  OMAPve_y_MDD_deceleration_typeNum/1 -> Bus Creator5/10  "OMAPve_y_MDD_deceleration_type_1"
  OMAPve_y_Powertrain_torquewheel_requestNum/1 -> Bus Creator/4  "OMAPve_y_Powertrain_torquewheel_request_1"
  OMAPve_y_AEB_Braking_progressNum/1 -> Bus Creator5/12  "OMAPve_y_AEB_Braking_progress_1"
  OMAPve_y_stAcvTqWhlPTPotReqNum/1 -> Bus Creator/6  "OMAPve_y_stAcvTqWhlPTPotReq_1"
  Bus Creator/1 -> EW_ISA_TSR_EMS/1  "EW_ISA_TSR_EMS"
  OMAPve_y_State_of_the_functionFARC_detNum/1 -> Bus Creator5/2  "OMAPve_y_State_of_the_functionFARC_det_1"
  OMAPve_y_MDD_Decelerationcontrol_requestNum/1 -> Bus Creator5/9  "OMAPve_y_MDD_Decelerationcontrol_request_1"
  OMAPve_y_Decel_RequestNum/1 -> Bus Creator5/11  "OMAPve_y_Decel_Request_1"
  Bus Creator5/1 -> EW_ISA_TSR_ESC/1  "EW_ISA_TSR_ESC"
  OMAPve_g_Coefficient_toregulate_EPSNum/1 -> Bus Creator10/3  "OMAPve_g_Coefficient_toregulate_EPS_2"
  OMAPve_g_Column_angle_setpoint3F2Num/1 -> Bus Creator10/4  "OMAPve_g_Column_angle_setpoint3F2_2"
  Bus Creator10/1 -> EW_ISA_TSR_EPS/1  "EW_ISA_TSR_EPS"
  OMAPve_y_Permit_to_know_if_LKA_or_LPA3F2Num/1 -> Bus Creator10/5  "OMAPve_y_Permit_to_know_if_LKA_or_LPA3F2_2"
  OMAPve_y_General_state_of_LKA_function3F2Num/1 -> Bus Creator10/2  "OMAPve_y_General_state_of_LKA_function3F2_2"
  OMAPve_y_Power_steering_power_cut3F2Num/1 -> Bus Creator10/1  "OMAPve_y_Power_steering_power_cut3F2_2"
  OMAPve_y_ADAS_ESCHoldReqNum/1 -> Bus Creator5/7  "OMAPve_y_ADAS_ESCHoldReq"
  OMAPve_y_ADAS_ESCDriveOffNum/1 -> Bus Creator5/6  "OMAPve_y_ADAS_ESCDriveOff"
  OMAPve_y_ADAS_ACCRequestEPBNum/1 -> Bus Creator5/13  "OMAPve_y_ADAS_ACCRequestEPB"
  Constant/1 -> Bus Creator1/31  "OMAPve_y_ADAS_LeftLEDWarningSt"
  Constant1/1 -> Bus Creator1/32  "OMAPve_y_ADAS_RighrLEDWarningSt"
  Bus Selector/1 -> Data Type Conversion5/1  "<EWWWve_y_SRR_SystemState_convert>"
  Bus Selector/2 -> Data Type Conversion1/1  "<EWWWve_y_BSD_SystemStateInfo_convert>"
  Bus Selector/3 -> Data Type Conversion14/1, Data Type Conversion2/1  "<EWWWve_y_LCW_M_SystemWorkingSt_convert>"
  Bus Selector/4 -> Data Type Conversion3/1, Data Type Conversion15/1  "<EWWWve_y_BSD_M_ErrorSt_convert>"
  Bus Selector/5 -> Data Type Conversion4/1  "<EWWWve_y_BSD_M_LCAWarning_convert>"
  Bus Selector/6 -> Data Type Conversion6/1  "<EWWWve_y_BSD_M_DoorOpenWarning_convert>"
  Bus Selector/7 -> Data Type Conversion7/1  "<EWWWve_y_BSD_M_RCTAWarning_convert>"
  Bus Selector/8 -> Data Type Conversion21/1, Data Type Conversion11/1  "<EWWWve_y_DOW_M_SystemWorkingSt_convert>"
  Bus Selector/9 -> Data Type Conversion22/1, Data Type Conversion12/1  "<EWWWve_y_RCTA_M_SystemWorkingSt_convert>"
  Bus Selector/11 -> Data Type Conversion16/1  "<EWWWve_y_BSD_S_LCAWarning_convert>"
  Bus Selector/12 -> Data Type Conversion19/1  "<EWWWve_y_BSD_S_DoorOpenWarning_convert>"
  Bus Selector/13 -> Data Type Conversion20/1  "<EWWWve_y_BSD_S_RCTAWarning_convert>"
  Bus Selector/14 -> Data Type Conversion23/1  "<EWWWve_y_SRR_LF_SystemStateInfo_convert>"
  Bus Selector/16 -> Data Type Conversion9/1, Data Type Conversion10/1  "<EWWWve_y_SRR_LF_ErrorSt_convert>"
  Bus Selector/17 -> Data Type Conversion18/1  "<EWWWve_y_SRR_LF_FCTAWarning_convert>"
  Bus Selector/18 -> Data Type Conversion17/1  "<EWWWve_y_SRR_RF_SystemStateInfo_convert>"
  Bus Selector/15 -> Data Type Conversion25/1, Data Type Conversion24/1  "<EWWWve_y_SRR_LF_FCTAWorkingSt_convert>"
  Bus Selector/19 -> Data Type Conversion8/1  "<EWWWve_y_SRR_RF_FCTAWarning_convert>"
  Bus Selector/10 -> Data Type Conversion13/1  "<EWWWve_y_BSD_S_SystemStateInfo_convert>"
  Data Type Conversion5/1 -> Bus Creator1/33  "OMAPve_y_ADAS_SRR_SystemState"
  Data Type Conversion1/1 -> Bus Creator1/34  "OMAPve_y_ADAS_BSD_SystemStInfo"
  Data Type Conversion2/1 -> Bus Creator1/35  "OMAPve_y_ADAS_BSD_LCWWorkingSt"
  Data Type Conversion3/1 -> Bus Creator1/37  "OMAPve_y_ADAS_BSD_ErrorSt"
  Data Type Conversion4/1 -> Bus Creator1/39  "OMAPve_y_ADAS_BSD_LCAWarning"
  Data Type Conversion6/1 -> Bus Creator1/40  "OMAPve_y_ADAS_BSD_DoorOpenWrn"
  Data Type Conversion7/1 -> Bus Creator1/41  "OMAPve_y_ADAS_BSD_RCTAWarning"
  Data Type Conversion8/1 -> Bus Creator1/57  "OMAPve_y_ADAS_SRR_RF_FCTAWrn"
  Data Type Conversion9/1 -> Bus Creator1/54  "OMAPve_y_ADAS_SRR-RF_ErrorSt"
  Data Type Conversion10/1 -> Bus Creator1/53  "OMAPve_y_ADAS_SRR-LF_ErrorSt"
  Data Type Conversion11/1 -> Bus Creator1/42  "OMAPve_y_ADAS_BSD_DOWWorkingSt"
  Data Type Conversion12/1 -> Bus Creator1/44  "OMAPve_y_ADAS_BSD_RCTAWorkingSt"
  Data Type Conversion13/1 -> Bus Creator1/46  "OMAPve_y_ADAS_BSD_S_SystStInfo"
  Data Type Conversion14/1 -> Bus Creator1/36  "OMAPve_y_ADAS_BSD_S_LCWWorkSt"
  Data Type Conversion15/1 -> Bus Creator1/38  "OMAPve_y_ADAS_BSD_S_ErrorSt"
  Data Type Conversion16/1 -> Bus Creator1/47  "OMAPve_y_ADAS_BSD_S_LCAWarning"
  Data Type Conversion17/1 -> Bus Creator1/56  "OMAPve_y_ADAS_SRR_RF_SystStInfo"
  Data Type Conversion18/1 -> Bus Creator1/55  "OMAPve_y_ADAS_SRR_LF_FCTAWrn"
  Data Type Conversion19/1 -> Bus Creator1/48  "OMAPve_y_ADAS_BSD_S_DoorOpenWrn"
  Data Type Conversion20/1 -> Bus Creator1/49  "OMAPve_y_ADAS_BSD_S_RCTAWarning"
  Data Type Conversion21/1 -> Bus Creator1/43  "OMAPve_y_ADAS_BSD_S_DOWWorkSt"
  Data Type Conversion22/1 -> Bus Creator1/45  "OMAPve_y_ADAS_BSD_S_RCTAWorkSt"
  Data Type Conversion23/1 -> Bus Creator1/50  "OMAPve_y_ADAS_SRR_LF_SystStInfo"
  Data Type Conversion24/1 -> Bus Creator1/51  "OMAPve_y_ADAS_SRR_LF_SystWorkSt"
  Data Type Conversion25/1 -> Bus Creator1/52  "OMAPve_y_ADAS_SRR_RF_SystWorkSt"
  OMAPve_y_ISA_Popup_textNum/1 -> Bus Creator1/2  "OMAPve_y_ISA_Popup_text_2"
  OMAPve_y_AEB_Fault_StatusNum/1 -> Bus Creator1/14  "OMAPve_y_AEB_Fault_Status_2"
  OMAPve_y_LDW_FlagNum/1 -> Bus Creator1/22  "OMAPve_y_LDW_Flag_2"
  OMAPve_y_HMI_Popup_StatusNum/1 -> Bus Creator1/20  "OMAPve_y_HMI_Popup_Status_2"
  OMAPve_y_LKA_Switch_StateNum/1 -> Bus Creator1/26  "OMAPve_y_LKA_Switch_State_2"
  OMAPve_y_Hands_off_warningNum/1 -> Bus Creator1/19  "OMAPve_y_Hands_off_warning_2"
  OMAPve_y_ACC_DesiredHeadway_Icon_BasicNum/1 -> Bus Creator1/7  "OMAPve_y_ACC_DesiredHeadway_Icon_Basic_2"
  OMAPve_y_ACC_Set_Speed_DisplayNum/1 -> Bus Creator1/9  "OMAPve_y_ACC_Set_Speed_Display_2"
  OMAPve_y_ACC_DesiredHeadway_DisplayNum/1 -> Bus Creator1/6  "OMAPve_y_ACC_DesiredHeadway_Display_2"
  OMAPve_y_AEB_Switch_StatusNum/1 -> Bus Creator1/15  "OMAPve_y_AEB_Switch_Status_2"
  OMAPve_y_ACC_Pop_Up_MessageNum/1 -> Bus Creator1/12  "OMAPve_y_ACC_Pop_Up_Message_2"
  OMAPve_y_ACC_Vehicle_Icon_DisplayNum/1 -> Bus Creator1/10  "OMAPve_y_ACC_Vehicle_Icon_Display_2"
  OMAPve_y_TARGET_POSITIONNum/1 -> Bus Creator1/18  "OMAPve_y_TARGET_POSITION_2"
  OMAPve_y_ADAS_ELKStsNum1/1 -> Bus Creator1/28  "OMAPve_y_ADAS_ELKSts_2"
  OMAPve_y_LDW_Status_DisplayNum/1 -> Bus Creator1/23  "OMAPve_y_LDW_Status_Display_2"
  OMAPve_y_ISA_StatusNum/1 -> Bus Creator1/4  "OMAPve_y_ISA_Status_2"
  OMAPve_y_TSR_Vision_Only_Sign_TypeNum/1 -> Bus Creator1/1  "OMAPve_y_TSR_Vision_Only_Sign_Type_2"
  OMAPve_y_ISA_Sign_TypeNum/1 -> Bus Creator1/3  "OMAPve_y_ISA_Sign_Type_2"
  OMAPve_y_LKA_Status_DisplayNum/1 -> Bus Creator1/25  "OMAPve_y_LKA_Status_Display_2"
  OMAPve_y_TJA_status_iconNum/1 -> Bus Creator1/30  "OMAPve_y_TJA_status_icon_2"
  OMAPve_y_ACC_Desired_Set_SpeedNum/1 -> Bus Creator1/8  "OMAPve_y_ACC_Desired_Set_Speed_2"
  OMAPve_y_LKA_action_indicationNum/1 -> Bus Creator1/27  "OMAPve_y_LKA_action_indication_2"
  OMAPve_y_AEB_tipsNum/1 -> Bus Creator1/16  "OMAPve_y_AEB_tips_2"
  OMAPve_y_Vehicle_Lane_DisplayNum/1 -> Bus Creator1/21  "OMAPve_y_Vehicle_Lane_Display_2"
  OMAPve_y_AEB_Alert_ReqNum/1 -> Bus Creator1/13  "OMAPve_y_AEB_Alert_Req_2"
  OMAPve_y_ACC_HMI_TgtDisp_FlagNum/1 -> Bus Creator1/17  "OMAPve_y_ACC_HMI_TgtDisp_Flag_2"
  OMAPve_y_LKA_Mode_from_CameraNum/1 -> Bus Creator1/24  "OMAPve_y_LKA_Mode_from_Camera_2"
  OMAPve_y_RVVACC_Vehiclespeed_request_typeNum/1 -> Bus Creator1/11  "OMAPve_y_RVVACC_Vehiclespeed_request_type_2"
  OMAPve_y_ISA_ValueNum/1 -> Bus Creator1/5  "OMAPve_y_ISA_Value_2"
  OMAPve_y_ICA_HMI_Txt_DispNum/1 -> Bus Creator1/29  "OMAPve_y_ICA_HMI_Txt_Disp_2"

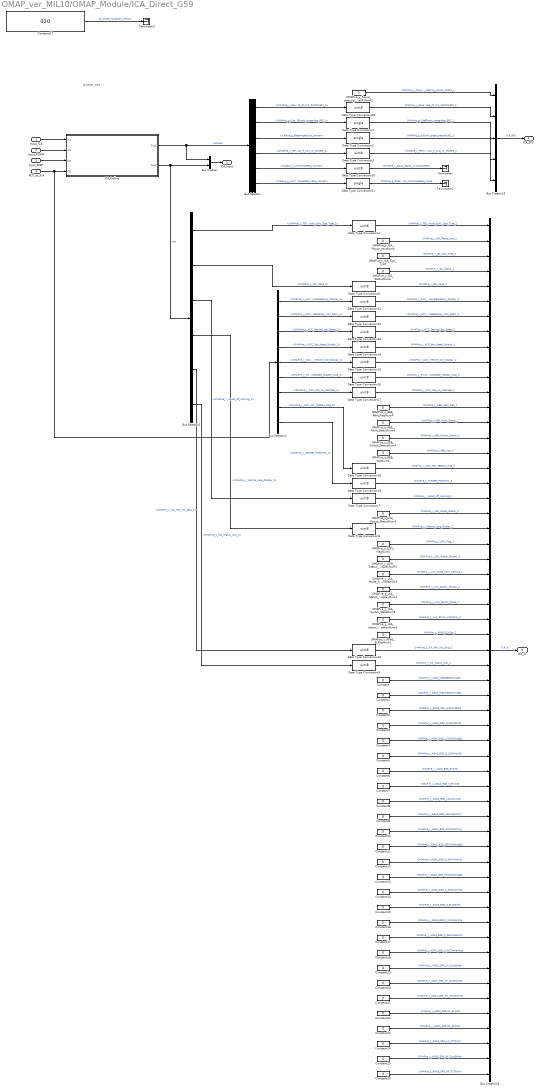
== system OMAP_ver_MIL10/OMAP_Module/ICA_Direct_G59 ==
  note: 配OMAP_G59
  Input_ICA : Inport
  Input_FDMM : Inport  Port=2
  Input_IMAP : Inport  Port=3
  ACC_to_ICA : Inport  Port=4
  Bus Creator : BusCreator  Inputs=2
  Bus Creator15 : BusCreator  Inputs=5
  Bus Creator24 : BusCreator  Inputs=57
  Bus Selector : BusSelector  OutputSignals=OMAPve_y_General_state_of_LKA_function3F2_2,OMAPve_g_Coefficient_toregulate_EPS_2,ICABve_g_SteerAngleCmd_convert,OMAPve_y_Permit_to_know_if_LKA_or_LPA3F2_2,ICABve_d_LKATorqueReq_convert,ICABve_g_LKATorqueReq_Value_convert
  Bus Selector1 : BusSelector  OutputSignals=OMAPve_y_TSR_Vision_Only_Sign_Type_2,OMAPve_y_ISA_Value_2,OMAPve_y_Hands_off_warning_2,OMAPve_y_Vehicle_Lane_Display_2,OMAPve_y_ICA_HMI_Txt_Disp_2,OMAPve_y_TJA_status_icon_2
  Bus Selector2 : BusSelector  OutputSignals=OMAPve_y_ACC_DesiredHeadway_Display_2,OMAPve_y_ACC_DesiredHeadway_Icon_Basic_2,OMAPve_y_ACC_Desired_Set_Speed_2,OMAPve_y_ACC_Set_Speed_Display_2,OMAPve_y_ACC_Vehicle_Icon_Display_2,OMAPve_y_RVVACC_Vehiclespeed_request_type_2,OMAPve_y_ACC_Pop_Up_Message_2,OMAPve_y_ACC_HMI_TgtDisp_Flag_2,OMAPve_y_TARGET_POSITION_2
  Constant{,1..26} (27 alike) : Constant  Value=0  OutDataTypeStr=uint8
  Constant27 : Constant  Value=020  OutDataTypeStr=uint16
  Data Type Conversion1 : DataTypeConversion  OutDataTypeStr=single
  Data Type Conversion{3..4,6..20,28} (18 alike) : DataTypeConversion  OutDataTypeStr=uint8
  Data Type Conversion2 : DataTypeConversion  OutDataTypeStr=single
  Data Type Conversion21 : DataTypeConversion  OutDataTypeStr=single
  ICA_Define : Subsystem
  OMAPve_y_ADAS_ELKStsNum1 : Constant  Value=0  OutDataTypeStr=uint8
  OMAPve_y_AEB_Alert_ReqNum4 : Constant  Value=0  OutDataTypeStr=uint8
  OMAPve_y_AEB_Fault_StatusNum4 : Constant  Value=0  OutDataTypeStr=uint8
  OMAPve_y_AEB_Switch_StatusNum4 : Constant  Value=0  OutDataTypeStr=uint8
  OMAPve_y_AEB_tipsNum4 : Constant  Value=0  OutDataTypeStr=uint8
  OMAPve_y_HMI_Popup_StatusNum4 : Constant  Value=0  OutDataTypeStr=uint8
  OMAPve_y_ISA_Popup_textNum6 : Constant  Value=0  OutDataTypeStr=uint8
  OMAPve_y_ISA_Sign_Type : Constant  Value=0  OutDataTypeStr=uint8
  OMAPve_y_ISA_StatusNum6 : Constant  Value=0  OutDataTypeStr=uint8
  OMAPve_y_LDW_FlagNum5 : Constant  Value=0  OutDataTypeStr=uint8
  OMAPve_y_LDW_Status_DisplayNum5 : Constant  Value=0  OutDataTypeStr=uint8
  OMAPve_y_LKA_Mode_from_CameraNum5 : Constant  Value=0  OutDataTypeStr=uint8
  OMAPve_y_LKA_Status_DisplayNum4 : Constant  Value=0  OutDataTypeStr=uint8
  OMAPve_y_LKA_Switch_StateNum5 : Constant  Value=0  OutDataTypeStr=uint8
  OMAPve_y_LKA_action_indicationNum4 : Constant  Value=0  OutDataTypeStr=uint8
  OMAPve_y_Power_steering_power_cut3F2Num2 : Constant  Value=0  OutDataTypeStr=uint8
  Terminator : Terminator
  Terminator1 : Terminator
  Terminator2 : Terminator
  ICA_EPS : Outport
  ICA_IC : Outport  Port=2
  ICA_Input : Outport  Port=3
  wires:
  OMAPve_y_AEB_Alert_ReqNum4/1 -> Bus Creator24/13  "OMAPve_y_AEB_Alert_Req_2"
  Data Type Conversion16/1 -> Bus Creator24/11  "OMAPve_y_RVVACC_Vehiclespeed_request_type_2"
  OMAPve_y_ISA_Popup_textNum6/1 -> Bus Creator24/2  "OMAPve_y_ISA_Popup_text_2"
  OMAPve_y_ISA_StatusNum6/1 -> Bus Creator24/4  "OMAPve_y_ISA_Status_2"
  Bus Selector1/3 -> Data Type Conversion7/1  "<OMAPve_y_Hands_off_warning_2>"
  Data Type Conversion12/1 -> Bus Creator24/7  "OMAPve_y_ACC_DesiredHeadway_Icon_Basic_2"
  Bus Selector1/2 -> Data Type Conversion6/1  "<OMAPve_y_ISA_Value_2>"
  Data Type Conversion14/1 -> Bus Creator24/9  "OMAPve_y_ACC_Set_Speed_Display_2"
  OMAPve_y_LDW_FlagNum5/1 -> Bus Creator24/22  "OMAPve_y_LDW_Flag_2"
  Bus Creator24/1 -> ICA_IC/1  "ICA_IC"
  OMAPve_y_AEB_tipsNum4/1 -> Bus Creator24/16  "OMAPve_y_AEB_tips_2"
  Bus Selector1/6 -> Data Type Conversion9/1  "<OMAPve_y_TJA_status_icon_2>"
  Data Type Conversion13/1 -> Bus Creator24/8  "OMAPve_y_ACC_Desired_Set_Speed_2"
  OMAPve_y_LKA_Status_DisplayNum4/1 -> Bus Creator24/25  "OMAPve_y_LKA_Status_Display_2"
  Data Type Conversion18/1 -> Bus Creator24/17  "OMAPve_y_ACC_HMI_TgtDisp_Flag_2"
  Data Type Conversion17/1 -> Bus Creator24/12  "OMAPve_y_ACC_Pop_Up_Message_2"
  OMAPve_y_LKA_Switch_StateNum5/1 -> Bus Creator24/26  "OMAPve_y_LKA_Switch_State_2"
  Data Type Conversion15/1 -> Bus Creator24/10  "OMAPve_y_ACC_Vehicle_Icon_Display_2"
  Bus Selector1/5 -> Data Type Conversion10/1  "<OMAPve_y_ICA_HMI_Txt_Disp_2>"
  OMAPve_y_LKA_Mode_from_CameraNum5/1 -> Bus Creator24/24  "OMAPve_y_LKA_Mode_from_Camera_2"
  OMAPve_y_LDW_Status_DisplayNum5/1 -> Bus Creator24/23  "OMAPve_y_LDW_Status_Display_2"
  OMAPve_y_AEB_Fault_StatusNum4/1 -> Bus Creator24/14  "OMAPve_y_AEB_Fault_Status_2"
  Bus Selector1/1 -> Data Type Conversion4/1  "<OMAPve_y_TSR_Vision_Only_Sign_Type_2>"
  OMAPve_y_HMI_Popup_StatusNum4/1 -> Bus Creator24/20  "OMAPve_y_HMI_Popup_Status_2"
  Bus Creator15/1 -> ICA_EPS/1  "ICA_EPS"
  Data Type Conversion11/1 -> Bus Creator24/6  "OMAPve_y_ACC_DesiredHeadway_Display_2"
  Data Type Conversion19/1 -> Bus Creator24/18  "OMAPve_y_TARGET_POSITION_2"
  OMAPve_y_AEB_Switch_StatusNum4/1 -> Bus Creator24/15  "OMAPve_y_AEB_Switch_Status_2"
  OMAPve_y_LKA_action_indicationNum4/1 -> Bus Creator24/27  "OMAPve_y_LKA_action_indication_2"
  Bus Selector1/4 -> Data Type Conversion8/1  "<OMAPve_y_Vehicle_Lane_Display_2>"
  Input_ICA/1 -> ICA_Define/1(In1)
  Input_IMAP/1 -> ICA_Define/3(In2)
  Input_FDMM/1 -> ICA_Define/2(In3)
  ACC_to_ICA/1 -> Bus Selector2/1, ICA_Define/4(In4)
  ICA_Define/2(Out2) -> Bus Creator/2, Bus Selector1/1  "HMI"
  Bus Creator/1 -> ICA_Input/1
  Data Type Conversion4/1 -> Bus Creator24/1  "OMAPve_y_TSR_Vision_Only_Sign_Type_2"
  OMAPve_y_ISA_Sign_Type/1 -> Bus Creator24/3  "OMAPve_y_ISA_Sign_Type_2"
  Data Type Conversion6/1 -> Bus Creator24/5  "OMAPve_y_ISA_Value_2"
  Data Type Conversion7/1 -> Bus Creator24/19  "OMAPve_y_Hands_off_warning_2"
  Data Type Conversion8/1 -> Bus Creator24/21  "OMAPve_y_Vehicle_Lane_Display_2"
  Data Type Conversion9/1 -> Bus Creator24/30  "OMAPve_y_TJA_status_icon_2"
  Data Type Conversion10/1 -> Bus Creator24/29  "OMAPve_y_ICA_HMI_Txt_Disp_2"
  Bus Selector2/1 -> Data Type Conversion11/1  "<OMAPve_y_ACC_DesiredHeadway_Display_2>"
  Bus Selector2/2 -> Data Type Conversion12/1  "<OMAPve_y_ACC_DesiredHeadway_Icon_Basic_2>"
  Bus Selector2/3 -> Data Type Conversion13/1  "<OMAPve_y_ACC_Desired_Set_Speed_2>"
  Bus Selector2/4 -> Data Type Conversion14/1  "<OMAPve_y_ACC_Set_Speed_Display_2>"
  Bus Selector2/5 -> Data Type Conversion15/1  "<OMAPve_y_ACC_Vehicle_Icon_Display_2>"
  Bus Selector2/6 -> Data Type Conversion16/1  "<OMAPve_y_RVVACC_Vehiclespeed_request_type_2>"
  Bus Selector2/7 -> Data Type Conversion17/1  "<OMAPve_y_ACC_Pop_Up_Message_2>"
  Bus Selector2/8 -> Data Type Conversion18/1  "<OMAPve_y_ACC_HMI_TgtDisp_Flag_2>"
  Bus Selector2/9 -> Data Type Conversion19/1  "<OMAPve_y_TARGET_POSITION_2>"
  OMAPve_y_ADAS_ELKStsNum1/1 -> Bus Creator24/28  "OMAPve_y_ADAS_ELKSts_2"
  Constant18/1 -> Bus Creator24/49  "OMAPve_y_ADAS_BSD_S_RCTAWarning"
  Constant5/1 -> Bus Creator24/36  "OMAPve_y_ADAS_BSD_S_LCWWorkSt"
  Constant4/1 -> Bus Creator24/35  "OMAPve_y_ADAS_BSD_LCWWorkingSt"
  Constant10/1 -> Bus Creator24/41  "OMAPve_y_ADAS_BSD_RCTAWarning"
  Constant6/1 -> Bus Creator24/37  "OMAPve_y_ADAS_BSD_ErrorSt"
  Constant22/1 -> Bus Creator24/53  "OMAPve_y_ADAS_SRR-LF_ErrorSt"
  Constant13/1 -> Bus Creator24/44  "OMAPve_y_ADAS_BSD_RCTAWorkingSt"
  Constant17/1 -> Bus Creator24/48  "OMAPve_y_ADAS_BSD_S_DoorOpenWrn"
  Constant3/1 -> Bus Creator24/34  "OMAPve_y_ADAS_BSD_SystemStInfo"
  Constant23/1 -> Bus Creator24/54  "OMAPve_y_ADAS_SRR-RF_ErrorSt"
  Constant/1 -> Bus Creator24/31  "OMAPve_y_ADAS_LeftLEDWarningSt"
  Constant7/1 -> Bus Creator24/38  "OMAPve_y_ADAS_BSD_S_ErrorSt"
  Constant16/1 -> Bus Creator24/47  "OMAPve_y_ADAS_BSD_S_LCAWarning"
  Constant15/1 -> Bus Creator24/46  "OMAPve_y_ADAS_BSD_S_SystStInfo"
  Constant12/1 -> Bus Creator24/43  "OMAPve_y_ADAS_BSD_S_DOWWorkSt"
  Constant11/1 -> Bus Creator24/42  "OMAPve_y_ADAS_BSD_DOWWorkingSt"
  Constant20/1 -> Bus Creator24/51  "OMAPve_y_ADAS_SRR_LF_SystWorkSt"
  Constant25/1 -> Bus Creator24/56  "OMAPve_y_ADAS_SRR_RF_SystStInfo"
  Constant2/1 -> Bus Creator24/33  "OMAPve_y_ADAS_SRR_SystemState"
  Constant24/1 -> Bus Creator24/55  "OMAPve_y_ADAS_SRR_LF_FCTAWrn"
  Constant26/1 -> Bus Creator24/57  "OMAPve_y_ADAS_SRR_RF_FCTAWrn"
  Constant1/1 -> Bus Creator24/32  "OMAPve_y_ADAS_RighrLEDWarningSt"
  Constant8/1 -> Bus Creator24/39  "OMAPve_y_ADAS_BSD_LCAWarning"
  Constant14/1 -> Bus Creator24/45  "OMAPve_y_ADAS_BSD_S_RCTAWorkSt"
  Constant9/1 -> Bus Creator24/40  "OMAPve_y_ADAS_BSD_DoorOpenWrn"
  Constant19/1 -> Bus Creator24/50  "OMAPve_y_ADAS_SRR_LF_SystStInfo"
  Constant21/1 -> Bus Creator24/52  "OMAPve_y_ADAS_SRR_RF_SystWorkSt"
  Data Type Conversion3/1 -> Bus Creator15/5  "OMAPve_y_Permit_to_know_if_LKA_or_LPA3F2_2"
  Bus Selector/5 -> Data Type Conversion20/1  "<ICABve_d_LKATorqueReq_convert>"
  Bus Selector/1 -> Data Type Conversion28/1  "<OMAPve_y_General_state_of_LKA_function3F2_2>"
  Bus Selector/4 -> Data Type Conversion3/1  "<OMAPve_y_Permit_to_know_if_LKA_or_LPA3F2_2>"
  Bus Selector/6 -> Data Type Conversion21/1  "<ICABve_g_LKATorqueReq_Value_convert>"
  Data Type Conversion20/1 -> Terminator/1  "OMAPve_y_DAS4_Status_LKATorqueReq"
  Bus Selector/2 -> Data Type Conversion1/1  "<OMAPve_g_Coefficient_toregulate_EPS_2>"
  OMAPve_y_Power_steering_power_cut3F2Num2/1 -> Bus Creator15/1  "OMAPve_y_Power_steering_power_cut3F2_2"
  Data Type Conversion1/1 -> Bus Creator15/3  "OMAPve_g_Coefficient_toregulate_EPS_2"
  Data Type Conversion28/1 -> Bus Creator15/2  "OMAPve_y_General_state_of_LKA_function3F2_2"
  Data Type Conversion21/1 -> Terminator1/1  "OMAPve_g_DAS4_Status_LKATorqueReq_Value"
  ICA_Define/1(Out1) -> Bus Selector/1, Bus Creator/1  "actuator"
  Bus Selector/3 -> Data Type Conversion2/1  "<ICABve_g_SteerAngleCmd_convert>"
  Data Type Conversion2/1 -> Bus Creator15/4  "OMAPve_g_Column_angle_setpoint3F2_2"
  Constant27/1 -> Terminator2/1  "ob_OMAP_ICAdirect_version"
